simulink model "fxpdemo_direct_form2"  (Simulink 7.6)
settings: Solver=FixedStepDiscrete  SolverMode=SingleTasking  StartTime=0.0  StopTime=200.0  FixedStep=1  RelTol=1e-3
Description:
  | Fixed-Point Direct Form Filter
  | 
  | It is straightforward to implement a direct form filter in fixed-point using fundamental
  | building blocks such as gain, delay, and sum.
settings Model: MinMaxOverflowLogging=MinMaxAndOverflow  Creator=The MathWorks Inc.  CovMetricSettings=d  ExtModeTrigMode=oneshot  ExtModeArmWhenConnect=off  ExtModeAutoUpdateStatusClock=off
settings DataIOCC: LimitDataPoints=off  SignalLoggingName=sigsOut
settings OptimizationCC: BooleanDataType=off  InlineInvariantSignals=on  InitFltsAndDblsToZero=on
settings DebuggingCC: SaveWithParameterizedLinksMsg=none  SignalResolutionControl=TryResolveAllWithWarning  SolverPrmCheckMsg=none  MultiTaskDSMMsg=warning  MultiTaskCondExecSysMsg=none  IntegerOverflowMsg=none  ParameterDowncastMsg=warning  ParameterOverflowMsg=warning  ParameterPrecisionLossMsg=none  StrictBusMsg=None
settings HardwareCC: TargetUnknown=on
settings RTWCC: IncludeERTFirstTime=on
settings GRTTargetCC: TargetFcnLib=ansi_tfl_tmw.mat

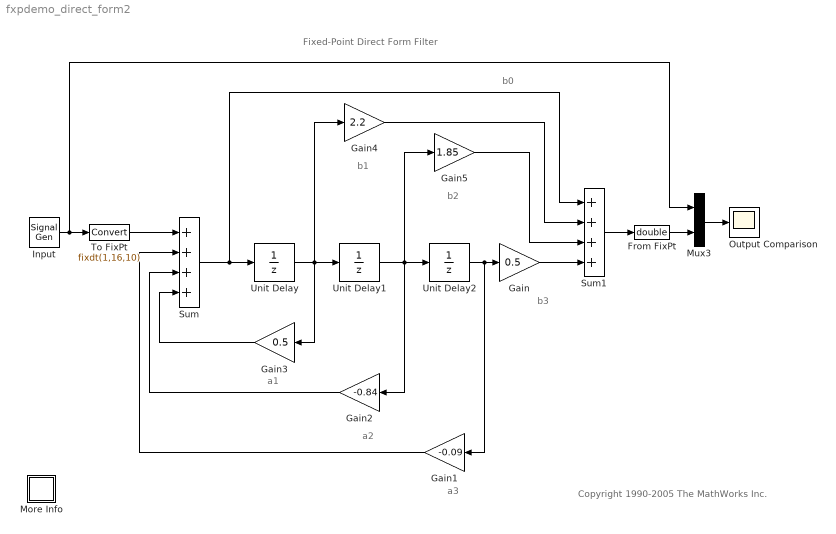
== system fxpdemo_direct_form2 ==
  note: b0
  note: b1
  note: b2
  note: b3
  note: a1
  note: a2
  note: a3
  note: Fixed-Point Direct Form Filter
  note: Copyright 1990-2005 The MathWorks Inc.
  From FixPt : DataTypeConversion  OutDataTypeStr=double
  Gain : Gain  Gain=0.5  ParamDataTypeStr=sfix( 16 )  OutDataTypeStr=fixdt(1,16,10)
  Gain1 : Gain  Gain=-0.09  ParamDataTypeStr=sfix( 16 )  OutDataTypeStr=fixdt(1,16,10)
  Gain2 : Gain  Gain=-0.84  ParamDataTypeStr=sfix( 16 )  OutDataTypeStr=fixdt(1,16,10)
  Gain3 : Gain  Gain=0.5  ParamDataTypeStr=sfix( 16 )  OutDataTypeStr=fixdt(1,16,10)
  Gain4 : Gain  Gain=2.2  ParamDataTypeStr=sfix( 16 )  OutDataTypeStr=fixdt(1,16,10)
  Gain5 : Gain  Gain=1.85  ParamDataTypeStr=sfix( 16 )  OutDataTypeStr=fixdt(1,16,10)
  Input : SignalGenerator  WaveForm=square  Frequency=0.005
  More Info : Subsystem
      settings: OpenFcn=showdemo(bdroot(gcs))
      mask Display: disp('?')
  Mux3 : Mux  Inputs=2
  Output Comparison : Scope
      settings: TickLabels=on  TimeRange=200  YMin=-8  YMax=10  SaveName=OutputComparison
  Sum : Sum  Inputs=++++  OutDataTypeStr=fixdt(1,16,10)
  Sum1 : Sum  Inputs=++++  OutDataTypeStr=fixdt(1,16,10)
  To FixPt : DataTypeConversion  OutDataTypeStr=fixdt(1,16,10)
  Unit Delay : UnitDelay  X0=0.0  SampleTime=1.0
  Unit Delay1 : UnitDelay  X0=0.0  SampleTime=1.0
  Unit Delay2 : UnitDelay  X0=0.0  SampleTime=1.0
  wires:
  Input/1 -> Mux3/1, To FixPt/1
  To FixPt/1 -> Sum/1
  Sum/1 -> Sum1/1, Unit Delay/1
  Gain3/1 -> Sum/4
  Unit Delay/1 -> Gain3/1, Gain4/1, Unit Delay1/1
  Gain2/1 -> Sum/3
  Unit Delay1/1 -> Unit Delay2/1, Gain5/1, Gain2/1
  Gain1/1 -> Sum/2
  Gain/1 -> Sum1/4
  Gain5/1 -> Sum1/3
  Gain4/1 -> Sum1/2
  Unit Delay2/1 -> Gain/1, Gain1/1
  Sum1/1 -> From FixPt/1
  From FixPt/1 -> Mux3/2
  Mux3/1 -> Output Comparison/1

== system fxpdemo_direct_form2/More Info ==
